simulink model "sys_ident"  (R2020b)
settings: Solver=VariableStepAuto  StartTime=0.0  StopTime=10.0  RelTol=1e-3
settings Model: Creator=a4327481  LastModifiedBy=a4327481

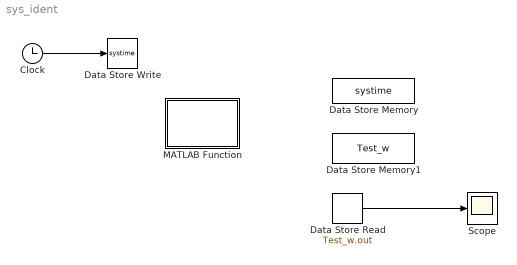
== system sys_ident ==
  Clock : Clock
  Data Store Memory : DataStoreMemory  DataStoreName=systime  ReadBeforeWriteMsg=warning  WriteAfterWriteMsg=warning  WriteAfterReadMsg=warning  InitialValue=systime  ShowAdditionalParam=off  OutDataTypeStr=double
  Data Store Memory1 : DataStoreMemory  DataStoreName=Test_w  ReadBeforeWriteMsg=warning  WriteAfterWriteMsg=warning  WriteAfterReadMsg=warning  InitialValue=Test_w  ShowAdditionalParam=off  OutDataTypeStr=Bus: Bus_Test_w
  Data Store Read : DataStoreRead  DataStoreName=Test_w  DataStoreElements=Test_w.out
  Data Store Write : DataStoreWrite  DataStoreName=systime
  MATLAB Function : MATLAB Function  TreatAsAtomicUnit=on
  Scope : Scope
  wires:
  Clock/1 -> Data Store Write/1
  Data Store Read/1 -> Scope/1

== matlab function sys_ident/MATLAB Function ==
  data: systime data_store_memory; Test_w data_store_memory
function fun
step_w();
end
